simulink model "Reaction_model_simulink_2_2"  (R2025b)
settings: Solver=VariableStepAuto  StartTime=0.0  StopTime=10.0  RelTol=1e-3
undefined symbols (not defined in the file or in its folder): Den, Jr, Num, Tc_max, wr_max
libraries: SignalEditorBlockLib x1
settings Model: Creator=flori  LastModifiedBy=flori

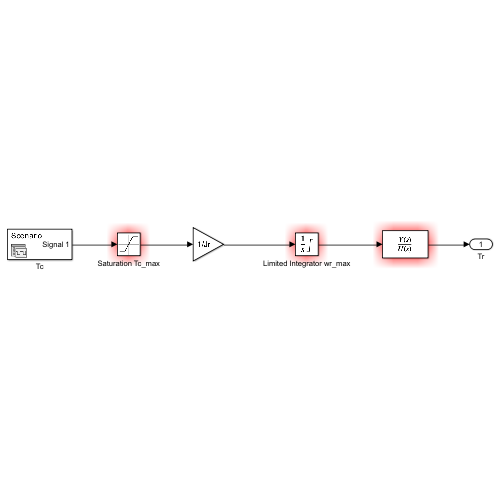
[thumbnail: Simulink's stored preview of the top-level diagram]
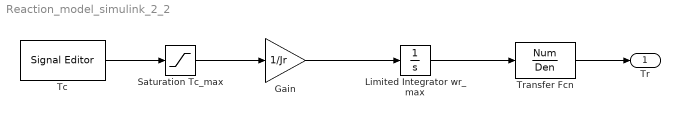
== system Reaction_model_simulink_2_2 ==
  Gain : Gain  Gain=1/Jr
  Limited Integrator wr_max : Integrator  LimitOutput=on  UpperSaturationLimit=wr_max  LowerSaturationLimit=-wr_max
  Saturation Tc_max : Saturate  UpperLimit=Tc_max  LowerLimit=-Tc_max
  Tc : SignalEditorBlockLib/Signal Editor  FileName=square signal.mat  ActiveScenario=Scenario  ActiveSignal=Signal 1  IsBus=off  OutputBusObjectStr=Bus: BusObject  SampleTime=0  ZeroCross=off  OutputAfterFinalValue=Setting to zero  Unit=inherit  PreserveSignalName=on  ApplySigPropsToAllScenarios=on  ApplySigPropsToAllSignals=off  SignalPropertySource=Dialog parameters
  Transfer Fcn : TransferFcn  Numerator=Num  Denominator=Den
  Tr : Outport
  wires:
  Saturation Tc_max/1 -> Gain/1
  Gain/1 -> Limited Integrator wr_max/1
  Limited Integrator wr_max/1 -> Transfer Fcn/1
  Tc/1 -> Saturation Tc_max/1
  Transfer Fcn/1 -> Tr/1
